simulink model "BESS_Harness"  (R2025b)
settings: Solver=VariableStepAuto  StartTime=0.0  StopTime=5  RelTol=1e-3
PostLoadFcn:
  | BESSParam
values from neighbouring files (symbols this model uses):
  bessVoltage = 1500    [BESSGFLParam.m]    (also in BESSGFMParam.m)
  gflInverter = struct    [BESSGFLParam.m]
  gfmInverter = struct    [BESSGFMParam.m]
  Ts = 5E-5    (= 5e-05)    [BESSGFLParam.m]    (also in BESSGFMParam.m; WindFarmParam.m)
undefined symbols (not defined in the file or in its folder): bessSystem, DiscIntNeverNeededParam, solar
libraries: eeGeneralControl x26, nesl_utility x26, ee_lib x16, simulink x12, fl_lib x10, eeTransforms x7, nesl_utility_internal x4, slpidlib x2, batteryecm_lib x2, simulink_extras x1, eePowerMeasurement x1, eePwmGenerator x1
(part 4 of 4)

== system BESS_Harness/BESS/Detailed/BESS Controller/Grid Forming/Current Limiting/CurrentLimitingMethod/currentSaturation/Compare ==
  u : Inport
  AND : Logic  IconShape=distinctive  AllPortsSameDT=off  OutDataTypeStr=boolean
  Compare To Constant : simulink/Logic and Bit Operations/Compare To Constant  relop=>  const=ctLimitDelayTime  OutDataTypeStr=boolean
  Compare To Zero : simulink/Logic and Bit Operations/Compare To Zero  relop=<=  OutDataTypeStr=boolean
  Data Type Conversion : DataTypeConversion  SaturateOnIntegerOverflow=off  RndMeth=Floor
  Data Type Conversion1 : DataTypeConversion  SaturateOnIntegerOverflow=off  RndMeth=Floor
  Discrete-Time Integrator : DiscreteIntegrator  IntegratorMethod=Integration: Backward Euler  ExternalReset=level  SampleTime=currentControlTs  LimitOutput=on  UpperSaturationLimit=ctLimitDelayTime*2  LowerSaturationLimit=0  ICPrevOutput=DiscIntNeverNeededParam  ICPrevScaledInput=DiscIntNeverNeededParam
  Out1 : Outport
  wires:
  Data Type Conversion1/1 -> AND/1, Discrete-Time Integrator/1, Discrete-Time Integrator/2
  Data Type Conversion/1 -> Out1/1
  Discrete-Time Integrator/1 -> Compare To Constant/1
  u/1 -> Compare To Zero/1
  Compare To Constant/1 -> AND/2
  Compare To Zero/1 -> Data Type Conversion1/1
  AND/1 -> Data Type Conversion/1

== system BESS_Harness/BESS/Detailed/BESS Controller/Grid Forming/Current Limiting/CurrentLimitingMethod/currentSaturation/If Action Subsystem ==
  Is : Inport
  Isd : Inport  Port=2
  Isq : Inport  Port=3
  Action Port : ActionPort  ActionPortLabel=if(u1 > 0)
  Constant : Constant  Value=maxSatCurrentLimit
  Divide : Product  Inputs=*/
  Product : Product
  Product1 : Product
  Idmax : Outport
  Iqmax : Outport  Port=2
  wires:
  Product/1 -> Iqmax/1
  Product1/1 -> Idmax/1
  Isq/1 -> Product/2
  Isd/1 -> Product1/1
  Divide/1 -> Product/1, Product1/2
  Is/1 -> Divide/2
  Constant/1 -> Divide/1

== system BESS_Harness/BESS/Detailed/BESS Controller/Grid Forming/Current Limiting/CurrentLimitingMethod/currentSaturation/If Action Subsystem1 ==
  Action Port : ActionPort  ActionPortLabel=else
  Constant3 : Constant  Value=0
  Constant4 : Constant  Value=0
  Idmax : Outport
  Iqmax : Outport  Port=2
  wires:
  Constant3/1 -> Idmax/1
  Constant4/1 -> Iqmax/1

== system BESS_Harness/BESS/Detailed/BESS Controller/Grid Forming/Grid Voltage Reactive Power Support/Modifying Reactive Power Reference/Changing the Power Reference/ActivePowerReference ==
  note: Ensure Pref sign is maintained
  Id : Inport
  Vd : Inport  Port=2
  Pref : Inport  Port=3
  Abs1 : Abs  SaturateOnIntegerOverflow=off
  Abs2 : Abs  SaturateOnIntegerOverflow=off
  Min : MinMax  Inputs=2
  Product : Product
  Product2 : Product
  Saturation : Saturate  UpperLimit=1  LowerLimit=-1
  Sign : Signum
  PrefNew : Outport
  wires:
  Saturation/1 -> PrefNew/1
  Vd/1 -> Product/2
  Abs2/1 -> Min/1
  Product2/1 -> Saturation/1
  Min/1 -> Product2/1
  Product/1 -> Abs2/1
  Abs1/1 -> Min/2
  Sign/1 -> Product2/2
  Id/1 -> Product/1
  Pref/1 -> Sign/1, Abs1/1

== system BESS_Harness/BESS/Detailed/BESS Controller/Grid Forming/Grid Voltage Reactive Power Support/Modifying Reactive Power Reference/Changing the Power Reference/EstimateIdForGivenIq ==
  Iq : Inport
  Add Constant1 : Bias  Bias=1*1  SaturateOnIntegerOverflow=off
  Gain : Gain  Gain=-1
  Gain3 : Gain  Gain=0.9
  Sqrt : Sqrt
  Square : Math  Operator=square
  Id : Outport
  wires:
  Iq/1 -> Square/1
  Add Constant1/1 -> Sqrt/1
  Sqrt/1 -> Gain3/1
  Gain/1 -> Add Constant1/1
  Gain3/1 -> Id/1
  Square/1 -> Gain/1

== system BESS_Harness/BESS/Detailed/BESS Controller/Grid Forming/Grid Voltage Reactive Power Support/Modifying Reactive Power Reference/Changing the Power Reference/EstimateIqForReactivePower ==
  note: Computing minimum reactive power as per GC0137
  Vmin : Inport
  Vd : Inport  Port=2
  Vs : Inport  Port=3
  Abs : Abs  SaturateOnIntegerOverflow=off
  Add : Sum
  Add Constant : Bias  Bias=1  SaturateOnIntegerOverflow=off
  GC0137 line slope : Gain  Gain=-1.4578
  Gain4 : Gain  Gain=1.5
  Saturation : Saturate  UpperLimit=1  LowerLimit=0
  Saturation1 : Saturate  UpperLimit=1  LowerLimit=-1
  Subtract : Sum  Inputs=+-
  Iq : Outport
  wires:
  Add Constant/1 -> Add/2
  Saturation/1 -> Iq/1
  Add/1 -> Saturation/1
  Vd/1 -> Subtract/2
  Vs/1 -> Abs/1
  Vmin/1 -> Subtract/1
  Gain4/1 -> Saturation1/1
  Saturation1/1 -> Add/1
  Subtract/1 -> Gain4/1
  GC0137 line slope/1 -> Add Constant/1
  Abs/1 -> GC0137 line slope/1

== system BESS_Harness/BESS/Detailed/BESS Controller/Grid Forming/Grid Voltage Reactive Power Support/Modifying Reactive Power Reference/Changing the Power Reference/ReactivePowerReference ==
  Vd : Inport
  Iq : Inport  Port=2
  Compute Power : Product
  Constant : Constant  Value=0.3
  Gain2 : Gain  Gain=1.05
  Switch : Switch  Criteria=u2 > Threshold  Threshold=0.3  SaturateOnIntegerOverflow=off  InputSameDT=off
  QrefNew : Outport
  wires:
  Switch/1 -> Compute Power/1
  Vd/1 -> Switch/1, Switch/2
  Iq/1 -> Gain2/1
  Constant/1 -> Switch/3
  Gain2/1 -> Compute Power/2
  Compute Power/1 -> QrefNew/1

== system BESS_Harness/BESS/Detailed/BESS Controller/Grid Forming/Measurement/Frequency Measurement/Frequency Measurement/If Action Subsystem ==
  V : Inport
  Time : Inport  Port=2
  Action Port : ActionPort  ActionPortLabel=if(u1 > 0.9)
  Constant1 : Constant  Value=initialFrequency
  Delay : Delay  DelayLength=1
  Delay1 : Delay  DelayLength=1
  Frequency estimation : Subsystem  TreatAsAtomicUnit=on
  Hit Crossing : HitCross
  Second-Order Filter : eeGeneralControl/Second-Order Filter  Commented=through  FilterType=Low-pass  fn=initialFrequency  Zeta=1  Ts=sampleTime  A0=0  Ph0=0  f0=0  b0=0
  Switch : Switch  Criteria=u2 > Threshold  Threshold=1  SaturateOnIntegerOverflow=off  InputSameDT=off
  Freq : Outport
  wires:
  Switch/1 -> Freq/1
  Constant1/1 -> Switch/3
  Frequency estimation/1(f) -> Switch/1
  Time/1 -> Frequency estimation/3(k), Delay1/1, Switch/2
  V/1 -> Second-Order Filter/1
  Delay/1 -> Frequency estimation/2(sk-1)
  Hit Crossing/1 -> Frequency estimation/Trigger
  Delay1/1 -> Frequency estimation/4(k-1)
  Second-Order Filter/1 -> Hit Crossing/1, Frequency estimation/1(sk), Delay/1

== system BESS_Harness/BESS/Detailed/BESS Controller/Grid Forming/Measurement/Frequency Measurement/Frequency Measurement/If Action Subsystem1 ==
  Action Port : ActionPort  ActionPortLabel=else
  Constant1 : Constant  Value=initialFrequency
  Out1 : Outport
  wires:
  Constant1/1 -> Out1/1

== system BESS_Harness/BESS/Detailed/BESS Controller/Grid Forming/Measurement/Frequency Measurement/Frequency Measurement/Postive Sequence ==
  abc : Inport
  Complex to Real-Imag : ComplexToRealImag
  Demux : Demux  Outputs=3
  Symmetrical-Components Transform : eeTransforms/Symmetrical-Components Transform  PowerInvariant=off
  Terminator : Terminator
  Terminator1 : Terminator
  Terminator2 : Terminator
  Transpose : Math  Operator=transpose
  posSeq : Outport
  wires:
  Demux/3 -> Terminator2/1
  Demux/2 -> Terminator1/1
  Complex to Real-Imag/2 -> Terminator/1
  abc/1 -> Transpose/1
  Demux/1 -> Complex to Real-Imag/1
  Complex to Real-Imag/1 -> posSeq/1
  Symmetrical-Components Transform/1 -> Demux/1
  Transpose/1 -> Symmetrical-Components Transform/1

== system BESS_Harness/BESS/Detailed/BESS Controller/Grid Forming/Power Control/ActivePowerControl/vsmControl/Damping Frequency ==
  fref : Inport
  ConstantFreqReference : Subsystem  VariantControl=constFreq
  WithFrequencyMeasurement : Subsystem  VariantControl=freqMeas
  fmeas : Outport

== system BESS_Harness/BESS/Detailed/BESS Controller/Grid Forming/Power Control/ActivePowerControl/vsmControl/Power Reference Selection ==
  cntrlflag : Inport
  Pref : Inport  Port=2
  fref : Inport  Port=3
  Wsm : Inport  Port=4
  If : If
  If Action Subsystem : Subsystem  TreatAsAtomicUnit=on
  If Action Subsystem1 : Subsystem  TreatAsAtomicUnit=on
  Merge : Merge
  Scope : Scope
  power : Outport
  wires:
  Wsm/1 -> [Wsm]
  Merge/1 -> power/1, Scope/1
  cntrlflag/1 -> If/1
  If/2 -> If Action Subsystem1/Action
  If Action Subsystem/1(Power) -> Merge/1
  [Wsm] -> If Action Subsystem/2(Wsm)
  fref/1 -> If Action Subsystem1/1(fref)
  [Wsm] -> If Action Subsystem1/2(Wsm)
  Pref/1 -> If Action Subsystem/1(Pref)
  If/1 -> If Action Subsystem/Action
  If Action Subsystem1/1(Power) -> Merge/2

== system BESS_Harness/BESS/Detailed/BESS Controller/Grid Forming/Power Control/ReactiveControl/Voltage  Reference Selection/If Action Subsystem ==
  note: Vs-delV
  Qref : Inport
  Qmeas : Inport  Port=2
  Action Port : ActionPort  ActionPortLabel=if(u1 > 0)
  Constant : Constant  Value=voltreference
  Gain : Gain  Gain=QVoltDroop
  Low-Pass Filter (Discrete or Continuous) : eeGeneralControl/Low-Pass Filter (Discrete or Continuous)  K=1  T=QVoltFilterTC  B=inf  A=-inf  init_option=Specify as parameter  x0=0  Ts=activePowerSampleTime
  Product1 : Product
  Scope : Scope
      settings: ActiveDisplayYMinimum=-0.00042  ActiveDisplayYMaximum=0.0007
  Scope1 : Scope  NumInputPorts=2
      settings: ActiveDisplayYMinimum=-0.71158  ActiveDisplayYMaximum=0.42604  DataLoggingVariableName=ScopeData5
  Sum : Sum  Inputs=|+-
  Sum1 : Sum  Inputs=|++
  Vd : Outport
  wires:
  Product1/1 -> Vd/1  "V"
  Sum1/1 -> Product1/1
  Sum/1 -> Gain/1
  Low-Pass Filter (Discrete or Continuous)/1 -> Sum/2
  Qref/1 -> Scope1/1, Sum/1
  Gain/1 -> Sum1/1, Scope/1
  Qmeas/1 -> Scope1/2, Low-Pass Filter (Discrete or Continuous)/1
  Constant/1 -> Sum1/2, Product1/2

== system BESS_Harness/BESS/Detailed/BESS Controller/Grid Forming/Power Control/ReactiveControl/Voltage  Reference Selection/If Action Subsystem1 ==
  note: Vs-delV
  Vref : Inport
  Vmeas : Inport  Port=2
  Action Port : ActionPort  ActionPortLabel=else
  Constant : Constant  Value=voltreference
  Gain : Gain  Gain=1e-3/QVoltDroop
  Low-Pass Filter (Discrete or Continuous) : eeGeneralControl/Low-Pass Filter (Discrete or Continuous)  K=1  T=QVoltFilterTC  B=inf  A=-inf  init_option=Specify as parameter  x0=0  Ts=activePowerSampleTime
  Product1 : Product
  Scope : Scope
      settings: ActiveDisplayYMinimum=8.18716  ActiveDisplayYMaximum=11.15581  DataLoggingVariableName=ScopeData11  DataLoggingSaveFormat=Array
  Scope1 : Scope
      settings: ActiveDisplayYMinimum=0.78014  ActiveDisplayYMaximum=0.78049  DataLoggingVariableName=ScopeData12  DataLoggingSaveFormat=Array
  Scope2 : Scope  NumInputPorts=2
      settings: ActiveDisplayYMinimum=0.83186  ActiveDisplayYMaximum=1.08242  DataLoggingVariableName=ScopeData13  DataLoggingSaveFormat=Array
  Sum : Sum  Inputs=|+-
  Sum1 : Sum  Inputs=|++
  Voltage : Outport
  wires:
  Sum1/1 -> Product1/2
  Product1/1 -> Scope/1, Voltage/1  "V"
  Sum/1 -> Gain/1
  Low-Pass Filter (Discrete or Continuous)/1 -> Scope1/1, Sum/2
  Constant/1 -> Sum1/2
  Vmeas/1 -> Low-Pass Filter (Discrete or Continuous)/1, Scope2/2
  Gain/1 -> Sum1/1
  Vref/1 -> Sum/1, Product1/1, Scope2/1

== system BESS_Harness/BESS/Detailed/BESS Controller/Grid Forming/Current Limiting/CurrentLimitingMethod/currentLimitAndVirtual/Current Saturation/Compare ==
  u : Inport
  Compare To Zero : simulink/Logic and Bit Operations/Compare To Zero  relop=<=  OutDataTypeStr=boolean
  Data Type Conversion : DataTypeConversion  SaturateOnIntegerOverflow=off  RndMeth=Floor
  Out1 : Outport
  wires:
  Data Type Conversion/1 -> Out1/1
  u/1 -> Compare To Zero/1
  Compare To Zero/1 -> Data Type Conversion/1

== system BESS_Harness/BESS/Detailed/BESS Controller/Grid Forming/Current Limiting/CurrentLimitingMethod/currentLimitAndVirtual/Current Saturation/If Action Subsystem ==
  Is : Inport
  Isd : Inport  Port=2
  Isq : Inport  Port=3
  maxI : Inport  Port=4
  Action Port : ActionPort
  Divide : Product  Inputs=*/
  Product : Product
  Product1 : Product
  Idmax : Outport
  Iqmax : Outport  Port=2
  wires:
  Product/1 -> Iqmax/1
  Product1/1 -> Idmax/1
  Isq/1 -> Product/2
  Isd/1 -> Product1/1
  Divide/1 -> Product/1, Product1/2
  Is/1 -> Divide/2
  maxI/1 -> Divide/1

== system BESS_Harness/BESS/Detailed/BESS Controller/Grid Forming/Current Limiting/CurrentLimitingMethod/currentLimitAndVirtual/Current Saturation/If Action Subsystem1 ==
  Action Port : ActionPort
  Constant3 : Constant  Value=0
  Constant4 : Constant  Value=0
  Idmax : Outport
  Iqmax : Outport  Port=2
  wires:
  Constant3/1 -> Idmax/1
  Constant4/1 -> Iqmax/1

== system BESS_Harness/BESS/Detailed/BESS Controller/Grid Forming/Measurement/Frequency Measurement/Frequency Measurement/If Action Subsystem/Frequency estimation ==
  sk : Inport
  sk-1 : Inport  Port=2
  k : Inport  Port=3
  k-1 : Inport  Port=4
  Trigger : TriggerPort  VariantControl=(inherit)  InitialTriggerSignalState=positive
  Add1 : Sum  Inputs=+-  OutDataTypeStr=double  AccumDataTypeStr=double  RndMeth=Convergent
  Add2 : Sum
  Constant : Constant
  Delay : Delay  DelayLength=1
  Delay1 : Delay  DelayLength=1
  Divide : Product  Inputs=*/  RndMeth=Ceiling
  Gain : Gain  Gain=2  ParamDataTypeStr=double  RndMeth=Convergent
  Gain2 : Gain  Gain=0.5
  MATLAB Function : MATLAB Function  TreatAsAtomicUnit=on
  f : Outport
  wires:
  sk-1/1 -> MATLAB Function/2(y2)
  sk/1 -> MATLAB Function/1(y1)
  k-1/1 -> MATLAB Function/4(x2)  "x1"
  k/1 -> MATLAB Function/3(x1)
  Delay/1 -> Add1/2
  Gain2/1 -> f/1
  Add2/1 -> Gain2/1
  Delay1/1 -> Add2/2
  Divide/1 -> Delay1/1, Add2/1
  MATLAB Function/1(x) -> Add1/1, Delay/1  "x1-y1/slope"
  Gain/1 -> Divide/2
  Constant/1 -> Divide/1
  Add1/1 -> Gain/1

== system BESS_Harness/BESS/Detailed/BESS Controller/Grid Forming/Power Control/ActivePowerControl/vsmControl/Damping Frequency/ConstantFreqReference ==
  fref : Inport
  Constant1 : Constant
  Terminator : Terminator
  fmeas : Outport
  wires:
  fref/1 -> Terminator/1
  Constant1/1 -> fmeas/1

== system BESS_Harness/BESS/Detailed/BESS Controller/Grid Forming/Power Control/ActivePowerControl/vsmControl/Damping Frequency/WithFrequencyMeasurement ==
  fref : Inport
  fmeas : Outport
  wires:
  fref/1 -> fmeas/1

== system BESS_Harness/BESS/Detailed/BESS Controller/Grid Forming/Power Control/ActivePowerControl/vsmControl/Power Reference Selection/If Action Subsystem ==
  note: Frequency difference power
  Pref : Inport
  Wsm : Inport  Port=2
  Action Port : ActionPort  ActionPortLabel=if(u1 > 0)
  Constant : Constant
  Gain6 : Gain  Gain=vsmFreqDroop
  Sum : Sum  Inputs=|+-
  Sum3 : Sum  Inputs=++|
  Power : Outport
  wires:
  Sum3/1 -> Power/1
  Constant/1 -> Sum/1
  Sum/1 -> Gain6/1
  Wsm/1 -> Sum/2
  Pref/1 -> Sum3/1  "Reference power"
  Gain6/1 -> Sum3/2

== system BESS_Harness/BESS/Detailed/BESS Controller/Grid Forming/Power Control/ActivePowerControl/vsmControl/Power Reference Selection/If Action Subsystem1 ==
  note: Frequency difference power
  fref : Inport
  Wsm : Inport  Port=2
  Action Port : ActionPort  ActionPortLabel=else
  Gain6 : Gain  Gain=vsmFreqDroop
  Scope : Scope
      settings: ActiveDisplayYMinimum=0.99966  ActiveDisplayYMaximum=1.00057  DataLoggingVariableName=ScopeData14
  Scope1 : Scope
      settings: DataLoggingVariableName=ScopeData15
  Sum : Sum  Inputs=|+-
  Power : Outport
  wires:
  Gain6/1 -> Power/1, Scope1/1
  fref/1 -> Sum/1
  Sum/1 -> Gain6/1
  Wsm/1 -> Sum/2, Scope/1

== stateflow chart BESS_Harness/BESS/Detailed/BESS Controller/Grid Forming/Current Limiting/CurrentLimitingMethod/currentLimitAndVirtual/CurrentLimitSelection ==
  state Mode1_VI_ON
    entry:
    noCurrentLimit  = 0;
    viCurrentLimit = 1;
    satCurrentLimit = 0;
    ismax= maxVICurrentLimit;
    exit:
    noCurrentLimit  = 0;
    viCurrentLimit = 1;
    satCurrentLimit = 0;
    ismax= maxVICurrentLimit;
  state Start_Mode
    entry:
    noCurrentLimit  = 1;
    viCurrentLimit = 0;
    satCurrentLimit = 0;
    ismax= maxSatCurrentLimit;
    exit:
    noCurrentLimit  = 1;
    viCurrentLimit = 0;
    satCurrentLimit = 0;
    ismax= maxSatCurrentLimit;
  state Mode2_CurrentSat_ON
    entry:
    noCurrentLimit  = 0;
    viCurrentLimit = 0;
    satCurrentLimit = 1;
    ismax= maxSatCurrentLimit;
    exit:
    noCurrentLimit  = 0;
    viCurrentLimit = 0;
    satCurrentLimit = 1;
    ismax= maxSatCurrentLimit;
  state Mode3_CurrentSat_ON
    entry:
    noCurrentLimit  = 0;
    viCurrentLimit = 0;
    satCurrentLimit = 1;
    ismax= 1.1*maxVICurrentLimit;
    exit:
    noCurrentLimit  = 0;
    viCurrentLimit = 0;
    satCurrentLimit = 1;
    ismax= 1.1*maxVICurrentLimit;
  Start_Mode -> Mode1_VI_ON : [Is>1]
  (junction 28) -> Mode1_VI_ON : after(currentControlTs*10, sec)[(Is<ismax) && (Is>1) ]
  Mode3_CurrentSat_ON -> (junction 28) [order 1]
  (default) -> Start_Mode
  Mode1_VI_ON -> Start_Mode [order 2] : [Is<1]
  Mode1_VI_ON -> Mode2_CurrentSat_ON [order 1] : after(0.5/powerFreq, sec)[(Is>=maxSatCurrentLimit)]
  (junction 26) -> Start_Mode
  Mode3_CurrentSat_ON -> Mode2_CurrentSat_ON [order 2] : after(0.5/powerFreq, sec)[(Is>ismax)]
  Mode2_CurrentSat_ON -> Mode3_CurrentSat_ON : after(currentSatTime, sec)[satCurrentLimit>0]
  Mode3_CurrentSat_ON -> (junction 26) [order 3] : [Is<1]
  data: Is input; ismax output; noCurrentLimit output; viCurrentLimit output; satCurrentLimit output; maxSatCurrentLimit parameter; maxVICurrentLimit parameter; currentControlTs parameter; currentSatTime parameter; powerFreq parameter

== matlab function BESS_Harness/BESS/Detailed/BESS Controller/Grid Forming/Measurement/Frequency Measurement/Frequency Measurement/If Action Subsystem/Frequency estimation/MATLAB Function ==
  data: y1 input; y2 input; x1 input; x output; x2 input
function x = fcn(y1,y2,x1,x2)
% Line equation between two points is y-y1=((y2-y1)/(x2-x1))*(x-x1). Here
% to to find the zero crossing instant substitute y = 0 and find x
slope = (y2-y1)/(x2-x1);
x = x1-y1/slope;
